simulink model "controladorVelho"  (R2018a)
settings: Solver=ode45  StartTime=0.0  StopTime=N  RelTol=1e-3
values from neighbouring files (symbols this model uses):
  R = 0.01    [init.m]
  x0 = x0barra + epsilon    [init.m]
undefined symbols (not defined in the file or in its folder): c, C, gama, phi, r
libraries: simulink x2, dspsrcs4 x1
settings Model: Creator=Raposo  LastModifiedBy=raposo
settings OptimizationCC: LifeSpan=inf
settings DebuggingCC: AllowSymbolicDim=off  SFExecutionAtInitializationDiag=none
settings HardwareCC: ProdBitPerSizeT=32  ProdBitPerPtrDiffT=32  ProdWordSize=32  ProdHWDeviceType=Specified
settings CodeAppCC: StateflowObjectComments=on

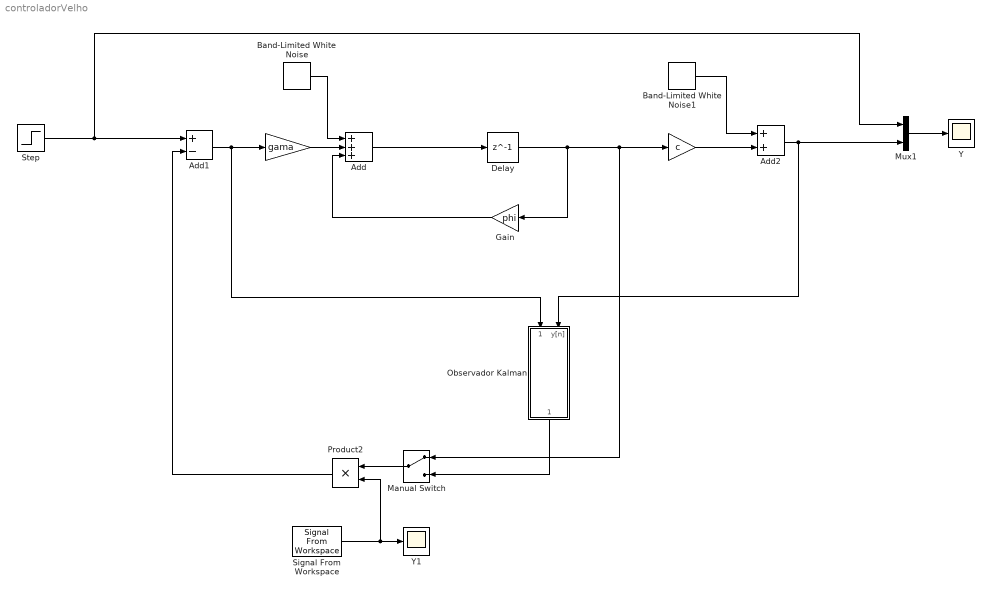
== system controladorVelho ==
  " " : Gain  Gain=c
  " " : Gain  Gain=gama
  Add : Sum  Inputs=+++
  Add1 : Sum  Inputs=+-
  Add2 : Sum
  Band-Limited White Noise : simulink/Sources/Band-Limited White Noise  Cov=[0.001]  Ts=0.1  seed=[23341]
  Band-Limited White Noise1 : simulink/Sources/Band-Limited White Noise  Cov=[0.001]  Ts=0.1  seed=[23341]
  Delay : Delay  DelayLength=1  InitialCondition=x0  SampleTime=[1,0]
  Gain : Gain  Gain=phi
  Manual Switch : ManualSwitch
  Mux1 : Mux  Inputs=2
  "Observador Kalman " : Subsystem
  Product2 : Product
  Signal From Workspace : dspsrcs4/Signal From Workspace  X=k  Ts=1  nsamps=1  OutputAfterFinalValue=Setting to zero  ignoreOrWarnInputAndFrameLengths=off  OutputFrames=on
  Step : Step  Time=5  SampleTime=0
  Y : Scope
  Y1 : Scope
  wires:
  Add/1 -> Delay/1
  Gain/1 -> Add/3
  Delay/1 -> Manual Switch/1, " "/1, Gain/1
  " "/1 -> Add/2
  " "/1 -> Add2/2
  Add2/1 -> "Observador Kalman "/2("y[n] "), Mux1/2
  Mux1/1 -> Y/1
  Step/1 -> Mux1/1, Add1/1
  Band-Limited White Noise/1 -> Add/1
  Band-Limited White Noise1/1 -> Add2/1
  Add1/1 -> "Observador Kalman "/1(u[n] 1), " "/1
  Signal From Workspace/1 -> Product2/2, Y1/1
  Product2/1 -> Add1/2
  Manual Switch/1 -> Product2/1
  "Observador Kalman "/1(X_hat_barra) -> Manual Switch/2

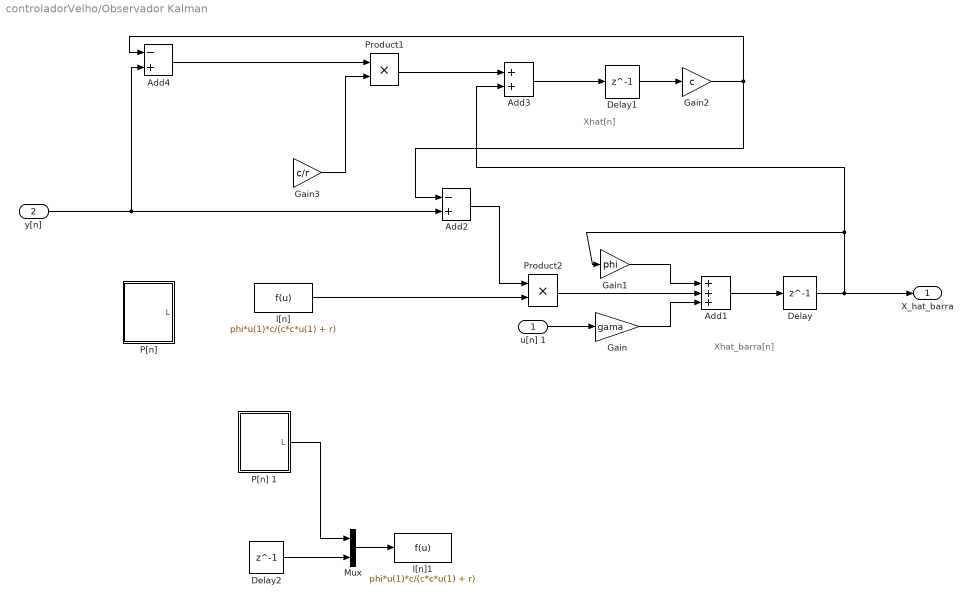
== system controladorVelho/Observador Kalman  ==
  note: Xhat_barra[n]
  note: Xhat[n]
  u[n] 1 : Inport
  "y[n] " : Inport  Port=2
  Add1 : Sum  Inputs=+++
  Add2 : Sum  Inputs=-+
  Add3 : Sum
  Add4 : Sum  Inputs=-+
  Delay : Delay  DelayLength=1  InitialCondition=0
  Delay1 : Delay  DelayLength=1  InitialCondition=0
  Delay2 : Delay  DelayLength=1  InitialCondition=0
  Gain : Gain  Gain=gama
  Gain1 : Gain  Gain=phi
  Gain2 : Gain  Gain=c
  Gain3 : Gain  Gain=c/r
  Mux : Mux  Inputs=2
  "P[n] " : Subsystem
  P[n] 1 : Subsystem
  Product1 : Product
  Product2 : Product
  l[n] : Fcn  Expr=phi*u(1)*c/(c*c*u(1) + r)
  l[n]1 : Fcn  Expr=phi*u(1)*c/(c*c*u(1) + r)
  X_hat_barra : Outport
  wires:
  "y[n] "/1 -> Add2/2, Add4/2
  Add1/1 -> Delay/1
  u[n] 1/1 -> Gain/1
  Gain/1 -> Add1/3
  Gain1/1 -> Add1/1
  Product2/1 -> Add1/2
  ? -> l[n]/1
  Add2/1 -> Product2/1
  Add3/1 -> Delay1/1
  Delay1/1 -> Gain2/1
  Delay/1 -> Add3/2, Gain1/1, X_hat_barra/1
  Gain2/1 -> Add2/1, Add4/1
  Add4/1 -> Product1/1
  Gain3/1 -> Product1/2
  ? -> Gain3/1
  Product1/1 -> Add3/1
  l[n]/1 -> Product2/2
  Mux/1 -> l[n]1/1
  P[n] 1/1(L) -> Mux/1
  Delay2/1 -> Mux/2

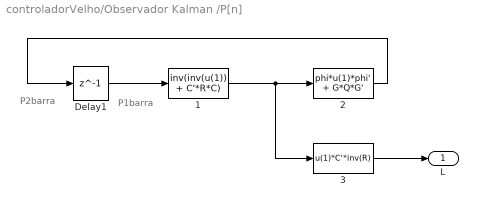
== system controladorVelho/Observador Kalman /P[n]  ==
  note: P2barra
  note: P1barra
  1 : Fcn  Expr=inv(inv(u(1)) + C'*R*C)
  2 : Fcn  Expr=phi*u(1)*phi' + G*Q*G'
  3 : Fcn  Expr=u(1)*C'*inv(R)
  Delay1 : Delay  DelayLength=1  InitialCondition=0
  L : Outport
  wires:
  Delay1/1 -> 1/1
  1/1 -> 3/1, 2/1
  2/1 -> Delay1/1
  3/1 -> L/1

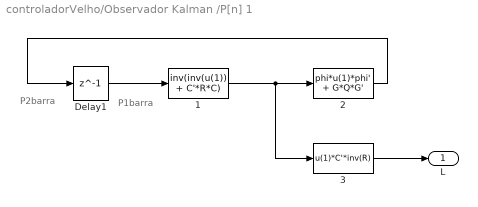
== system controladorVelho/Observador Kalman /P[n] 1 ==
  note: P2barra
  note: P1barra
  1 : Fcn  Expr=inv(inv(u(1)) + C'*R*C)
  2 : Fcn  Expr=phi*u(1)*phi' + G*Q*G'
  3 : Fcn  Expr=u(1)*C'*inv(R)
  Delay1 : Delay  DelayLength=1  InitialCondition=0
  L : Outport
  wires:
  Delay1/1 -> 1/1
  1/1 -> 3/1, 2/1
  2/1 -> Delay1/1
  3/1 -> L/1
